simulink model "kitticopter_closedloop"  (R2025b)
settings: Solver=ode45  StartTime=0.0  StopTime=400  MaxStep=0.1  RelTol=1e-3
values from neighbouring files (symbols this model uses):
  A = 14.1208    [circuit_model.m]    (also in closed_sweep.m; controller_simualtion_result.m; open_loop.m)
  k = find(tp > t0_fit & vel >= V63, 1, 'first')    [velocity_position_plots.m]
  T = readtable(dataFile)    [open_loop.m]    (also in velocity_position_plots.m)
undefined symbols (not defined in the file or in its folder): dV, Kp, Vh, Xstep
settings Model: Creator=MTMTAD006  LastModifiedBy=MTMTAD006

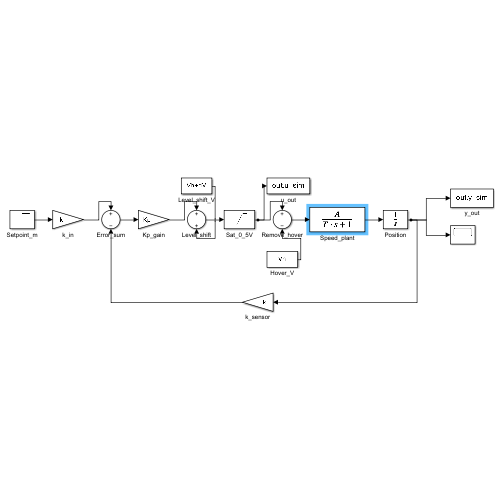
[thumbnail: Simulink's stored preview of the top-level diagram]
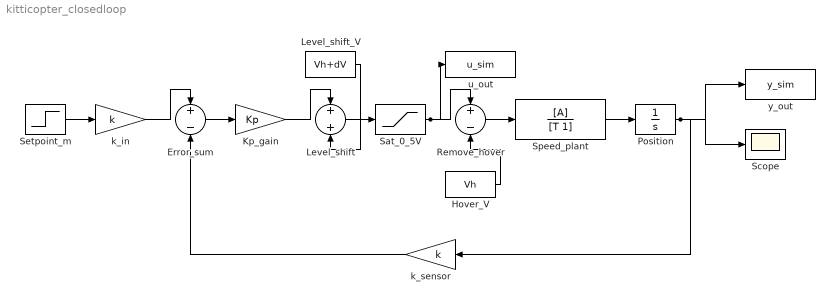
== system kitticopter_closedloop ==
  Error_sum : Sum  Inputs=+-
  Hover_V : Constant  Value=Vh
  Kp_gain : Gain  Gain=Kp
  Level_shift : Sum
  Level_shift_V : Constant  Value=Vh+dV
  Position : Integrator
  Remove_hover : Sum  Inputs=+-
  Sat_0_5V : Saturate  UpperLimit=5  LowerLimit=0
  Scope : Scope
      settings: ActiveDisplayYMinimum=-0.97838731328712947  ActiveDisplayYMaximum=8.8054858195841668
  Setpoint_m : Step  Time=0  After=Xstep  SampleTime=0
  Speed_plant : TransferFcn  Numerator=[A]  Denominator=[T 1]
  k_in : Gain  Gain=k
  k_sensor : Gain  Gain=k
  u_out : ToWorkspace  VariableName=u_sim  SaveFormat=Timeseries  SampleTime=-1
  y_out : ToWorkspace  VariableName=y_sim  SaveFormat=Timeseries  SampleTime=-1
  wires:
  Setpoint_m/1 -> k_in/1
  k_in/1 -> Error_sum/1
  Error_sum/1 -> Kp_gain/1
  Kp_gain/1 -> Level_shift/1
  Level_shift_V/1 -> Level_shift/2
  Level_shift/1 -> Sat_0_5V/1
  Sat_0_5V/1 -> Remove_hover/1, u_out/1
  Hover_V/1 -> Remove_hover/2
  Remove_hover/1 -> Speed_plant/1
  Speed_plant/1 -> Position/1
  Position/1 -> k_sensor/1, y_out/1, Scope/1
  k_sensor/1 -> Error_sum/2
